simulink library "SimFly_RC"  (R2015b)
settings: Solver=VariableStepAuto  StartTime=0.0  StopTime=10.0  RelTol=1e-3
settings Model: Creator=mocherma  LastModifiedBy=mocherma

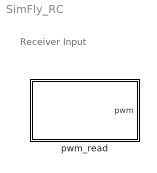
== system SimFly_RC ==
  note: Receiver Input
  pwm_read : MATLAB Function  TreatAsAtomicUnit=on  mask(SimFly PWMIN){pwm_sample=-1}
      mask prompts: pwm_sample "Sample Time"
      mask help: 8 Receiver Inputs in micro seconds

== matlab function SimFly_RC/pwm_read ==
  settings: updateMethod=DISCRETE  sampleTime=pwm_sample
  data: pwm output
function pwm =  pwm_read
% Simulink Arduino Block Driver Library for Autocode Generation
 % 
 % This file is part of the Simulink Arduino Block Driver Library 
 % for Autocode Generation with Simulink
 %
 % This Library is free software: you can redistribute it and/or modify
 % it under the terms of the GNU General Public License as published by
 % the Free Software Foundation, either version 3 of the License, or
 % (at your option) any later version.
 %
 % This Library is distributed in the hope that it will be useful,
 % but WITHOUT ANY WARRANTY; without even the implied warranty of
 % MERCHANTABILITY or FITNESS FOR A PARTICULAR PURPOSE.  See the
 % GNU General Public License for more details.
 %
 % You should have received a copy of the GNU General Public License
 % along with this Library.  If not, see
 % <http://www.gnu.org/licenses/>.
 %
%
%PURPOSE: Reads PWM signals from receiver
%AUTHOR: Marcell Mocher
%DATE: 10.6.2016
%VERSION: 0.1 V Fist build
%Input: -
%Output:    pwm[8*1](single) =  pwm signal micro seconds
%           status[8*1] (single) = status flag if channel is working
%Info: This drive requires function call triggered simuluink functions in
% order to work
%Requires:  _pwmin_attach
%           _pwmin_step
persistent init_flag pwm_out


if strcmp(coder.target,'rtw')
    if isempty(init_flag)
        init_flag = 1;
        pwm_out = uint16(zeros(8,1));
        coder.ceval('_pwmin_attach',uint8(8));
    end 
    
    pwm_read = uint16(zeros(8,1));
    status_read = uint16(zeros(8,1));
    coder.ceval('_pwmin_step',uint8(8),coder.ref(pwm_read),coder.ref(status_read));
    
    for i = 1:8
        if pwm_read(i) > 0
        pwm_out(i) =  pwm_read(i);
        end
    end
    pwm = pwm_out;
else
    pwm = uint16(zeros(8,1));
end
